simulink model "Task_21"  (R2022b)
settings: Solver=VariableStepAuto  StartTime=0.0  StopTime=10.0  RelTol=1e-3
libraries: simulink x1
settings Model: Creator=Abanob_Sameh  LastModifiedBy=Abanob_Sameh

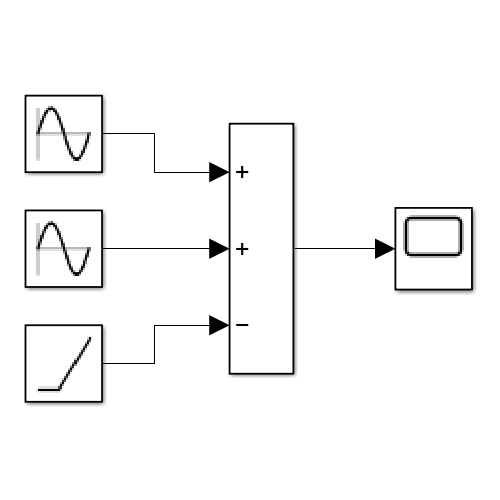
[thumbnail: Simulink's stored preview of the top-level diagram]
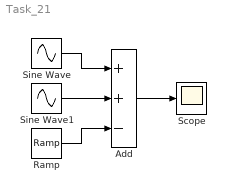
== system Task_21 ==
  Add : Sum  Inputs=++-
  Ramp : simulink/Sources/Ramp  slope=1  start=0  InitialOutput=0
  Scope : Scope
  Sine Wave : Sin  Frequency=5  SampleTime=0
  Sine Wave1 : Sin  Frequency=3  SampleTime=0
  wires:
  Add/1 -> Scope/1
  Sine Wave/1 -> Add/1
  Sine Wave1/1 -> Add/2
  Ramp/1 -> Add/3
